simulink model "MIMOsimulink_model"  (R2017b)
settings: Solver=VariableStepAuto  StartTime=0.0  StopTime=270  RelTol=1e-3
settings Model: Creator=ladislav  LastModifiedBy=ladislav

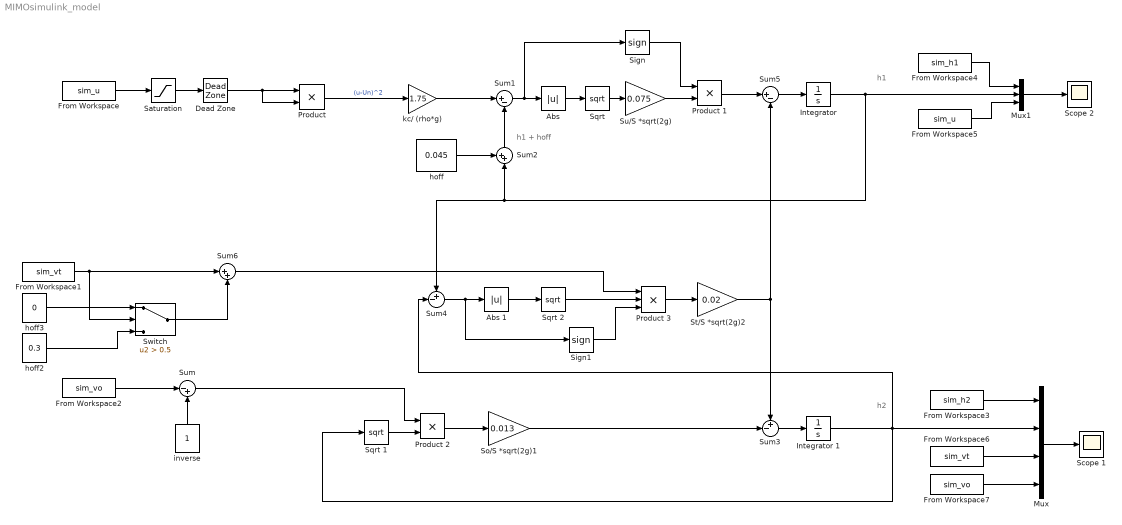
== system MIMOsimulink_model ==
  note: h1
  note: h1 + hoff
  note: h2
  " hoff" : Constant  Value=0.045
  " hoff2" : Constant  Value=0.3
  " hoff3" : Constant  Value=0
  " inverse" : Constant
  "Abs " : Abs
  Abs 1 : Abs
  "Dead Zone " : DeadZone  LowerValue=0  UpperValue=0.05  SaturateOnIntegerOverflow=on
  From Workspace : FromWorkspace  VariableName=sim_u  SampleTime=0
  From Workspace1 : FromWorkspace  VariableName=sim_vt  SampleTime=0
  From Workspace2 : FromWorkspace  VariableName=sim_vo  SampleTime=0
  From Workspace3 : FromWorkspace  VariableName=sim_h2  SampleTime=0
  From Workspace4 : FromWorkspace  VariableName=sim_h1  SampleTime=0
  From Workspace5 : FromWorkspace  VariableName=sim_u  SampleTime=0
  From Workspace6 : FromWorkspace  VariableName=sim_vt  SampleTime=0
  From Workspace7 : FromWorkspace  VariableName=sim_vo  SampleTime=0
  "Integrator " : Integrator  InitialCondition=-0.045  LimitOutput=on  UpperSaturationLimit=0.71  LowerSaturationLimit=-0.045
  Integrator 1 : Integrator  LimitOutput=on  UpperSaturationLimit=0.71  LowerSaturationLimit=0
  Mux : Mux
  Mux1 : Mux  Inputs=3
  "Product " : Product
  Product 1 : Product
  Product 2 : Product
  Product 3 : Product  Inputs=3
  "Saturation " : Saturate  UpperLimit=1
  Scope 1 : Scope
  Scope 2 : Scope
  Sign : Signum
  Sign1 : Signum
  So/S *sqrt(2g)1 : Gain  Gain=0.013
  "Sqrt " : Sqrt  SaturateOnIntegerOverflow=on
  Sqrt 1 : Sqrt  SaturateOnIntegerOverflow=on
  Sqrt 2 : Sqrt  SaturateOnIntegerOverflow=on
  St/S *sqrt(2g)2 : Gain  Gain=0.02
  Su/S *sqrt(2g) : Gain  Gain=0.075
  Sum : Sum  Inputs=|-+
  Sum1 : Sum  Inputs=|+-
  Sum2 : Sum  Inputs=++|
  Sum3 : Sum  Inputs=+-|
  Sum4 : Sum  Inputs=+-|
  Sum5 : Sum  Inputs=|+-
  Sum6 : Sum  Inputs=|++
  Switch : Switch  Criteria=u2 > Threshold  Threshold=0.5
  kc/ (rho*g) : Gain  Gain=1.75
  wires:
  "Dead Zone "/1 -> "Product "/2, "Product "/1
  "Product "/1 -> kc/ (rho*g)/1  "(u-Un)^2"
  "Sqrt "/1 -> Su/S *sqrt(2g)/1
  Sum2/1 -> Sum1/2
  " hoff"/1 -> Sum2/1
  "Integrator "/1 -> Sum4/1, Sum2/2, Mux1/2
  Integrator 1/1 -> Sum4/2, Mux/2, Sqrt 1/1
  kc/ (rho*g)/1 -> Sum1/1
  Sum1/1 -> Sign/1, "Abs "/1
  "Abs "/1 -> "Sqrt "/1
  Sign/1 -> Product 1/1
  Su/S *sqrt(2g)/1 -> Product 1/2
  Sqrt 1/1 -> Product 2/2
  Product 2/1 -> So/S *sqrt(2g)1/1
  Sum3/1 -> Integrator 1/1
  So/S *sqrt(2g)1/1 -> Sum3/2
  Abs 1/1 -> Sqrt 2/1
  Sum4/1 -> Sign1/1, Abs 1/1
  Product 3/1 -> St/S *sqrt(2g)2/1
  St/S *sqrt(2g)2/1 -> Sum5/2, Sum3/1
  Product 1/1 -> Sum5/1
  Sum5/1 -> "Integrator "/1
  Sign1/1 -> Product 3/3
  Sqrt 2/1 -> Product 3/2
  From Workspace3/1 -> Mux/1
  Mux/1 -> Scope 1/1
  Mux1/1 -> Scope 2/1
  From Workspace4/1 -> Mux1/1
  From Workspace2/1 -> Sum/1
  " inverse"/1 -> Sum/2
  From Workspace5/1 -> Mux1/3
  From Workspace6/1 -> Mux/3
  From Workspace7/1 -> Mux/4
  Sum/1 -> Product 2/1
  From Workspace/1 -> "Saturation "/1
  Sum6/1 -> Product 3/1
  From Workspace1/1 -> Switch/2, Sum6/1
  " hoff3"/1 -> Switch/1
  " hoff2"/1 -> Switch/3
  Switch/1 -> Sum6/2
  "Saturation "/1 -> "Dead Zone "/1
